simulink model "lab_roomreverbsimulation"  (R2018a)
settings: Solver=VariableStepAuto  StartTime=0.0  StopTime=2  RelTol=1e-3
libraries: dspvision x2
settings Model: Creator=lw199  LastModifiedBy=lw199

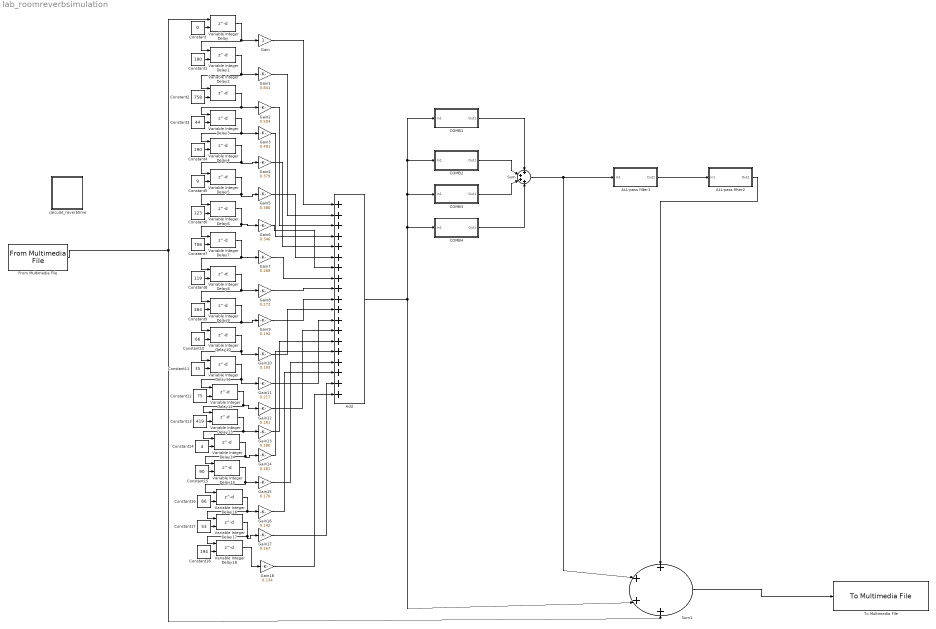
== system lab_roomreverbsimulation ==
  "ALL-pass filter1 " : Subsystem
  "ALL-pass filter2 " : Subsystem
  Add : Sum  Inputs=+++++++++++++++++++
  COMB1 : Subsystem
  COMB2 : Subsystem
  COMB3 : Subsystem
  "COMB4 " : Subsystem
  Constant : Constant  Value=0
  Constant1 : Constant  Value=190
  Constant10 : Constant  Value=66
  Constant11 : Constant  Value=35
  Constant12 : Constant  Value=75
  Constant13 : Constant  Value=419
  Constant14 : Constant  Value=4
  Constant15 : Constant  Value=90
  Constant16 : Constant  Value=66
  Constant17 : Constant  Value=53
  Constant18 : Constant  Value=194
  Constant2 : Constant  Value=758
  Constant3 : Constant  Value=44
  Constant4 : Constant  Value=190
  Constant5 : Constant  Value=9
  Constant6 : Constant  Value=123
  Constant7 : Constant  Value=706
  Constant8 : Constant  Value=119
  Constant9 : Constant  Value=384
  From Multimedia File : dspvision/From Multimedia File  inputFilename=E:\大二下课件\DSP\实验\2018212601-唐宏京-DSP 创新实验\DATA\audio.wav  loop=on  numPlays=2  outputStreams=Audio only  videoDataType=single  audioDataType=double  inheritSampleTime=on  userDefinedSampleTime=1/30  noAudioOutput=off  isIntensityVideo=off  fourcc=RGB  colorVideoFormat=One multidimensional signal  outputEOF=off  dataOrg=Column-major  audioFrameSize=1  computeAudioFrameSize=off  outSamplingMode=Sample based
      settings: SourceProductBaseCode=VP
  Gain : Gain
  Gain1 : Gain  Gain=0.841
  Gain10 : Gain  Gain=0.193
  Gain11 : Gain  Gain=0.217
  Gain12 : Gain  Gain=0.181
  Gain13 : Gain  Gain=0.180
  Gain14 : Gain  Gain=0.181
  Gain15 : Gain  Gain=0.176
  Gain16 : Gain  Gain=0.142
  Gain17 : Gain  Gain=0.167
  Gain18 : Gain  Gain=0.134
  Gain2 : Gain  Gain=0.504
  Gain3 : Gain  Gain=0.491
  Gain4 : Gain  Gain=0.379
  Gain5 : Gain  Gain=0.380
  Gain6 : Gain  Gain=0.346
  Gain7 : Gain  Gain=0.289
  Gain8 : Gain  Gain=0.272
  Gain9 : Gain  Gain=0.192
  Sum : Sum  Inputs=++++
  Sum1 : Sum  Inputs=++++
  To Multimedia File : dspvision/To Multimedia File  outputFilename=E:\大二下课件\DSP\实验\2018212601-唐宏京-DSP 创新实验\reverbed_audio_roomsize5-5-2.wav  streamSelection=Audio only  videoCompressor=None (uncompressed)  audioCompressor=None (uncompressed)  imagePorts=Separate color signals  fileType=WAV  audioDatatype=16-bit integer  fourcc=RGB  videoQuality=75  mj2000CompFactor=10
      settings: SourceProductName=Computer Vision System Toolbox  SourceProductBaseCode=VP
  Variable Integer Delay{,1..18} (19 alike) : Delay  DelayLengthSource=Input port  DelayLength=0
      settings: InputPortMap=u0,p1
  "calculat_reverbtime " : Subsystem
      mask Display: image('functions.bmp')
  wires:
  COMB1/1(Out1) -> Sum/1
  COMB2/1(Out1) -> Sum/2
  COMB3/1(Out1) -> Sum/3
  "COMB4 "/1(Out1) -> Sum/4
  Sum/1 -> Sum1/2, "ALL-pass filter1 "/1(In1)
  "ALL-pass filter1 "/1(Out1) -> "ALL-pass filter2 "/1(In1)
  Add/1 -> Sum1/3, COMB1/1(In1), COMB2/1(In1), COMB3/1(In1), "COMB4 "/1(In1)
  Constant/1 -> Variable Integer Delay/2
  Constant1/1 -> Variable Integer Delay1/2
  Constant2/1 -> Variable Integer Delay2/2
  From Multimedia File/1 -> Sum1/4, Variable Integer Delay/1
  Variable Integer Delay/1 -> Variable Integer Delay1/1, Gain/1
  Variable Integer Delay1/1 -> Variable Integer Delay2/1, Gain1/1
  Constant3/1 -> Variable Integer Delay3/2
  Variable Integer Delay2/1 -> Gain2/1, Variable Integer Delay3/1
  Constant4/1 -> Variable Integer Delay4/2
  Variable Integer Delay3/1 -> Gain3/1, Variable Integer Delay4/1
  Constant5/1 -> Variable Integer Delay5/2
  Variable Integer Delay4/1 -> Variable Integer Delay5/1, Gain4/1
  Constant6/1 -> Variable Integer Delay6/2
  Variable Integer Delay5/1 -> Variable Integer Delay6/1, Gain5/1
  Constant7/1 -> Variable Integer Delay7/2
  Variable Integer Delay6/1 -> Gain6/1, Variable Integer Delay7/1
  Constant8/1 -> Variable Integer Delay8/2
  Variable Integer Delay7/1 -> Gain7/1, Variable Integer Delay8/1
  Constant9/1 -> Variable Integer Delay9/2
  Variable Integer Delay8/1 -> Gain8/1, Variable Integer Delay9/1
  Constant10/1 -> Variable Integer Delay10/2
  Variable Integer Delay9/1 -> Gain9/1, Variable Integer Delay10/1
  Constant11/1 -> Variable Integer Delay11/2
  Variable Integer Delay10/1 -> Gain10/1, Variable Integer Delay11/1
  Constant12/1 -> Variable Integer Delay12/2
  Variable Integer Delay11/1 -> Gain11/1, Variable Integer Delay12/1
  Constant13/1 -> Variable Integer Delay13/2
  Variable Integer Delay12/1 -> Gain12/1, Variable Integer Delay13/1
  Constant14/1 -> Variable Integer Delay14/2
  Variable Integer Delay13/1 -> Gain13/1, Variable Integer Delay14/1
  Constant15/1 -> Variable Integer Delay15/2
  Variable Integer Delay14/1 -> Variable Integer Delay15/1, Gain14/1
  Constant16/1 -> Variable Integer Delay16/2
  Variable Integer Delay15/1 -> Variable Integer Delay16/1, Gain15/1
  Constant17/1 -> Variable Integer Delay17/2
  Variable Integer Delay16/1 -> Gain16/1, Variable Integer Delay17/1
  Constant18/1 -> Variable Integer Delay18/2
  Variable Integer Delay17/1 -> Variable Integer Delay18/1, Gain17/1
  Variable Integer Delay18/1 -> Gain18/1
  Gain/1 -> Add/1
  Gain1/1 -> Add/2
  Gain2/1 -> Add/3
  Gain3/1 -> Add/4
  Gain4/1 -> Add/5
  Gain5/1 -> Add/6
  Gain6/1 -> Add/7
  Gain7/1 -> Add/8
  Gain8/1 -> Add/9
  Gain9/1 -> Add/10
  Gain10/1 -> Add/11
  Gain11/1 -> Add/12
  Gain12/1 -> Add/13
  Gain13/1 -> Add/14
  Gain14/1 -> Add/15
  Gain15/1 -> Add/16
  Gain16/1 -> Add/17
  Gain17/1 -> Add/18
  Gain18/1 -> Add/19
  "ALL-pass filter2 "/1(Out1) -> Sum1/1
  Sum1/1 -> To Multimedia File/1

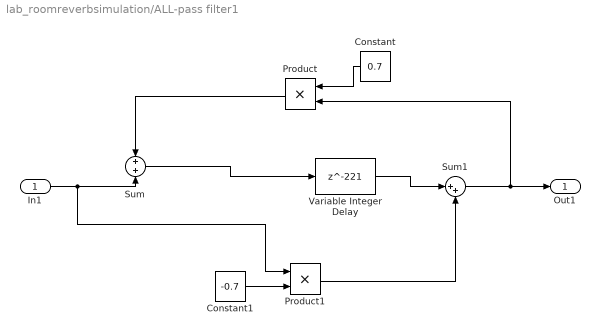
== system lab_roomreverbsimulation/ALL-pass filter1  ==
  In1 : Inport
  Constant : Constant  Value=0.7
  Constant1 : Constant  Value=-0.7
  Product : Product
  Product1 : Product
  Sum : Sum
  Sum1 : Sum  Inputs=|++
  Variable Integer Delay : Delay  DelayLength=221
  Out1 : Outport
  wires:
  In1/1 -> Product1/1, Sum/2
  Sum1/1 -> Product/2, Out1/1
  Constant1/1 -> Product1/2
  Constant/1 -> Product/1
  Product1/1 -> Sum1/2
  Sum/1 -> Variable Integer Delay/1
  Variable Integer Delay/1 -> Sum1/1
  Product/1 -> Sum/1

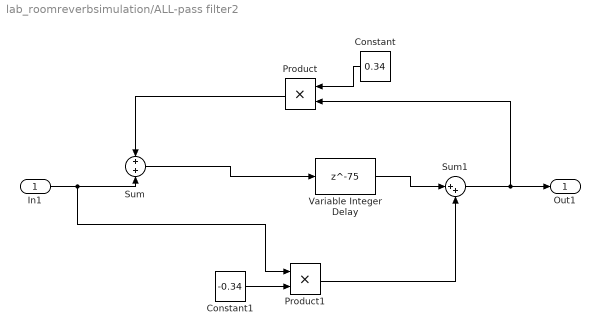
== system lab_roomreverbsimulation/ALL-pass filter2  ==
  In1 : Inport
  Constant : Constant  Value=0.34
  Constant1 : Constant  Value=-0.34
  Product : Product
  Product1 : Product
  Sum : Sum
  Sum1 : Sum  Inputs=|++
  Variable Integer Delay : Delay  DelayLength=75
  Out1 : Outport
  wires:
  In1/1 -> Product1/1, Sum/2
  Sum1/1 -> Product/2, Out1/1
  Constant1/1 -> Product1/2
  Constant/1 -> Product/1
  Product1/1 -> Sum1/2
  Sum/1 -> Variable Integer Delay/1
  Variable Integer Delay/1 -> Sum1/1
  Product/1 -> Sum/1

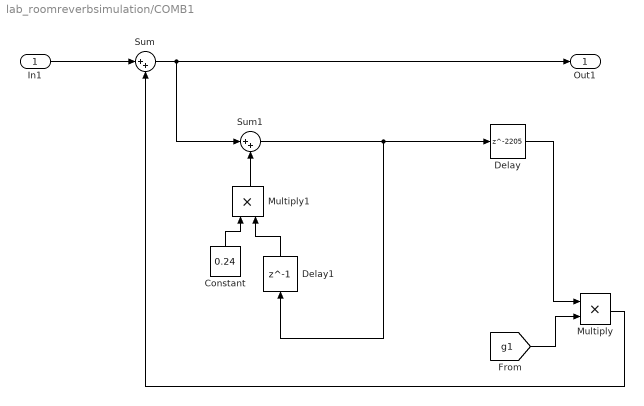
== system lab_roomreverbsimulation/COMB1 ==
  In1 : Inport
  Constant : Constant  Value=0.24
  Delay : Delay  DelayLength=2205  InitialCondition=0
  Delay1 : Delay  DelayLength=1  InitialCondition=0
  Multiply : Product
  Multiply1 : Product
  Sum : Sum  Inputs=|++
  Sum1 : Sum  Inputs=|++
  Out1 : Outport
  wires:
  Sum/1 -> Sum1/1, Out1/1
  Delay/1 -> Multiply/1
  In1/1 -> Sum/1
  [g1] -> Multiply/2
  Multiply/1 -> Sum/2
  Sum1/1 -> Delay1/1, Delay/1
  Multiply1/1 -> Sum1/2
  Constant/1 -> Multiply1/1
  Delay1/1 -> Multiply1/2

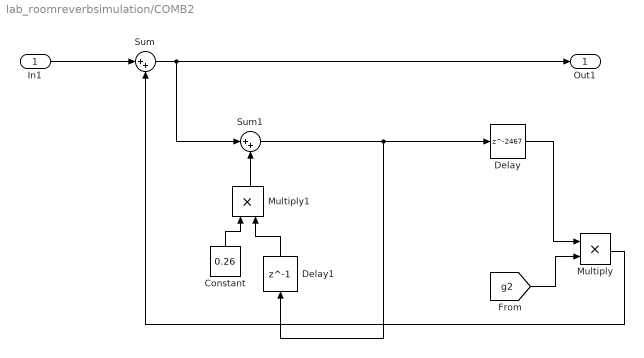
== system lab_roomreverbsimulation/COMB2 ==
  In1 : Inport
  Constant : Constant  Value=0.26
  Delay : Delay  DelayLength=2467  InitialCondition=0
  Delay1 : Delay  DelayLength=1  InitialCondition=0
  Multiply : Product
  Multiply1 : Product
  Sum : Sum  Inputs=|++
  Sum1 : Sum  Inputs=|++
  Out1 : Outport
  wires:
  Sum/1 -> Sum1/1, Out1/1
  Delay/1 -> Multiply/1
  In1/1 -> Sum/1
  [g2] -> Multiply/2
  Multiply/1 -> Sum/2
  Sum1/1 -> Delay1/1, Delay/1
  Multiply1/1 -> Sum1/2
  Constant/1 -> Multiply1/1
  Delay1/1 -> Multiply1/2

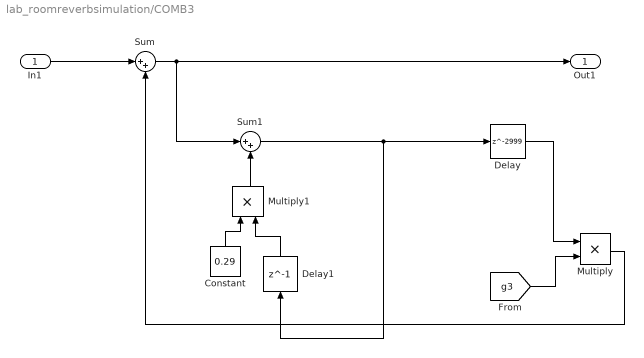
== system lab_roomreverbsimulation/COMB3 ==
  In1 : Inport
  Constant : Constant  Value=0.29
  Delay : Delay  DelayLength=2999  InitialCondition=0
  Delay1 : Delay  DelayLength=1  InitialCondition=0
  Multiply : Product
  Multiply1 : Product
  Sum : Sum  Inputs=|++
  Sum1 : Sum  Inputs=|++
  Out1 : Outport
  wires:
  Sum/1 -> Sum1/1, Out1/1
  Delay/1 -> Multiply/1
  In1/1 -> Sum/1
  [g3] -> Multiply/2
  Multiply/1 -> Sum/2
  Sum1/1 -> Delay1/1, Delay/1
  Multiply1/1 -> Sum1/2
  Constant/1 -> Multiply1/1
  Delay1/1 -> Multiply1/2

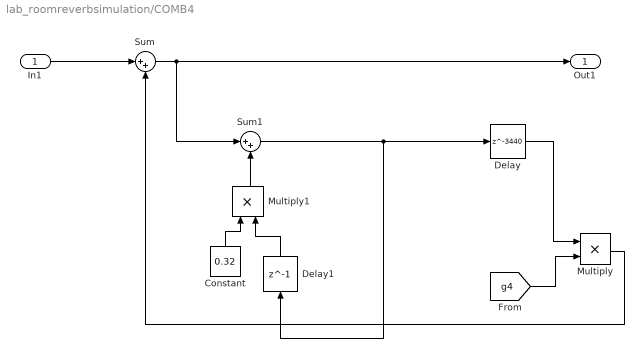
== system lab_roomreverbsimulation/COMB4  ==
  In1 : Inport
  Constant : Constant  Value=0.32
  Delay : Delay  DelayLength=3440  InitialCondition=0
  Delay1 : Delay  DelayLength=1  InitialCondition=0
  Multiply : Product
  Multiply1 : Product
  Sum : Sum  Inputs=|++
  Sum1 : Sum  Inputs=|++
  Out1 : Outport
  wires:
  Sum/1 -> Sum1/1, Out1/1
  Delay/1 -> Multiply/1
  In1/1 -> Sum/1
  [g4] -> Multiply/2
  Multiply/1 -> Sum/2
  Sum1/1 -> Delay1/1, Delay/1
  Multiply1/1 -> Sum1/2
  Constant/1 -> Multiply1/1
  Delay1/1 -> Multiply1/2

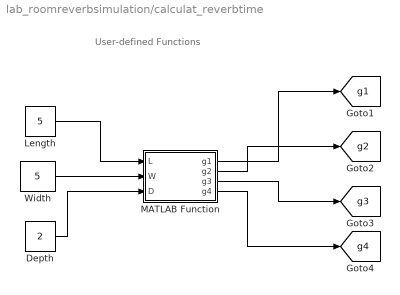
== system lab_roomreverbsimulation/calculat_reverbtime  ==
  note: User-defined Functions
  Depth : Constant  Value=2
  Length : Constant  Value=5
  MATLAB Function : MATLAB Function  TreatAsAtomicUnit=on
  Width : Constant  Value=5
  tag scope: g1=global, g2=global, g3=global, g4=global
  wires:
  Length/1 -> MATLAB Function/1(L)
  Width/1 -> MATLAB Function/2(W)
  Depth/1 -> MATLAB Function/3(D)
  MATLAB Function/1(g1) -> [g1]
  MATLAB Function/2(g2) -> [g2]
  MATLAB Function/3(g3) -> [g3]
  MATLAB Function/4(g4) -> [g4]

== matlab function lab_roomreverbsimulation/calculat_reverbtime /MATLAB Function ==
  data: L input; W input; D input; g1 output; g2 output; g3 output; g4 output
function [g1,g2,g3,g4]= reverbtime(L,W,D)
%generate the parameters in relevence of reverb time
%L:length W:width D:depth
%calculate T_60: reverb time,based on Sabine eqation
v=L*W*D;
s=L*W*2+L*D*2+W*D*2;
T_60 = (0.16*v)/(0.1*s);

%generate a: attenuation coefficent for lp filter
a=[0.24 0.26 0.29 0.32]

%calculate g:feedback coeficent,based on Moorer model
g1=(1-0.366/T_60)*(1-a(1,1));
g2=(1-0.366/T_60)*(1-a(1,2));
g3=(1-0.366/T_60)*(1-a(1,1));
g4=(1-0.366/T_60)*(1-a(1,1));
